simulink model "Model1"  (R2021a)
settings: Solver=VariableStepAuto  StartTime=0.0  StopTime=10.0  RelTol=1e-3
settings Model: Creator=ameya  LastModifiedBy=ameya

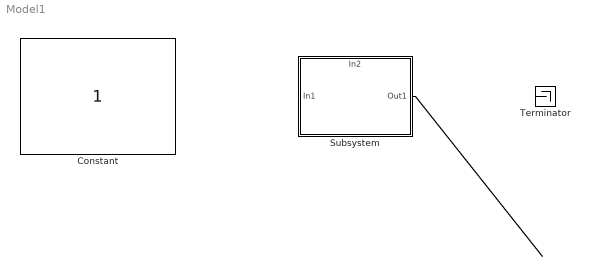
== system Model1 ==
  Constant : Constant
  Subsystem : Subsystem
      settings: PortSchema="{\"entries\":[{\"content\":{\"sides\":[{\"content\":{\"connectorIds\":[\"In1\"]},\"type\":\"ConnectorPlacement.EquallySpacedRectSide\",\"uuid\":\"679f6c73-f7f5-4400-8c1d-0750732bf36a\"},{\"content\":{\"connectorIds\":[\"Out1\"],\"side\":\"RIGHT\"},\"type\":\"ConnectorPlacement.EquallySpacedRectSide\",\"uuid\":\"e37b9cab-8b43-46dc-81ae-632f83d803c5\"},{\"content\":{\"connectorIds\":[\"In2\"],\"side\":\"TOP\"},\"type\":\"ConnectorPlacement.EquallySpacedRectSide\",\"uuid\":\"820a4bdc-041d-4dd1-a0d2-b6f3f577a394\"}]},\"type\":\"ConnectorPlacement.EquallySpacedConnector\",\"uuid\":\"b76735f2-df35-48d5-8bd7-ea83bcd5193a\"}],\"packageUris\":[\"http://schema.mathworks.com/mf0/Connector/R2020b\"],\"version\":\"1.0\"}"
  Terminator : Terminator
  wires:
  ? -> Subsystem/2(In2)
  ? -> Terminator/1
  Subsystem/1(Out1) -> ?

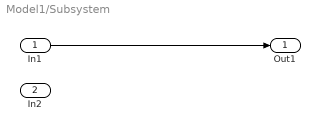
== system Model1/Subsystem ==
  In1 : Inport
  In2 : Inport  Port=2
  Out1 : Outport
  wires:
  In1/1 -> Out1/1
